simulink model "ex01_trafficA"  (R2020b)
settings: Solver=VariableStepAuto  StartTime=0.0  StopTime=60  RelTol=1e-3
model workspace (MAT data in the model file):
  courseObject.course = 'stateflow'
  courseObject.chapter = 3
  courseObject.lesson = 3
  courseObject.section = 1
  courseObject.task = 1
settings Model: NumberOfSteps=3  EnablePacing=on  PacingRate=3  Creator=gb  LastModifiedBy=19255551
settings DataIOCC: SaveTime=off

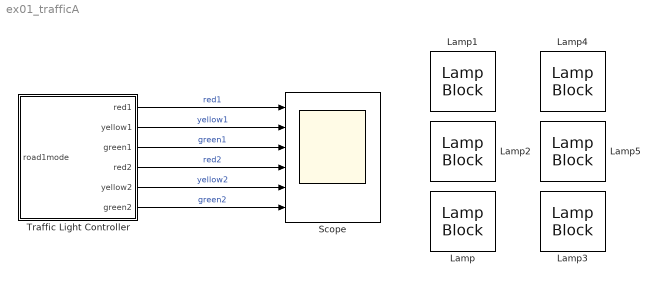
== system ex01_trafficA ==
  Lamp{,1..5} (6 alike) : LampBlock
  Scope : Scope  NumInputPorts=6
  Traffic Light Controller : Stateflow chart  TreatAsAtomicUnit=on
  wires:
  Traffic Light Controller/3(green1) -> Scope/3  "green1"
  Traffic Light Controller/1(red1) -> Scope/1  "red1"
  Traffic Light Controller/2(yellow1) -> Scope/2  "yellow1"
  Traffic Light Controller/4(red2) -> Scope/4  "red2"
  Traffic Light Controller/5(yellow2) -> Scope/5  "yellow2"
  Traffic Light Controller/6(green2) -> Scope/6  "green2"

== stateflow chart ex01_trafficA/Traffic Light Controller ==
  state Road1Go
    entry:
    green1 = 1;
    red2 = 1;
    red1 = 0;
    yellow2 = 0;
  state Road1Wait
    entry:
    green1 = 0;
    yellow1 = 1;
    red2 = 1;
  state Start1
    entry:
    red1 = 1;
    red2 = 1;
    yellow1 = 0;
    yellow2 = 0;
  state Road2Wait
    entry:
    green2 = 0;
    yellow2 = 1;
    red1 = 1;
  state Road2Go
    entry:
    yellow1 = 0;
    red1 = 1;
    green2 = 1;
    red2 = 0;
  (default) -> Start1
  Start1 -> Road1Go : after(5,sec)
  Road1Go -> Road1Wait : after(8,sec)
  Road1Wait -> Road2Go : after(2,sec)
  Road2Wait -> Road1Go : after(2,sec)
  Road2Go -> Road2Wait : after(8,sec)
  data: red1 output; yellow1 output; green1 output; red2 output; yellow2 output; green2 output; road1mode input
